simulink model "Sensing_Circuit_Test"  (R2020b)
settings: Solver=FixedStepAuto  StartTime=0.0  StopTime=10.0  FixedStep=1e-3  RelTol=1e-3  EnableMultiTasking=on
undefined symbols (not defined in the file): D0, D1, D13, D3, D6, PTA1, PTC16, PTC17, PTC2, PTD1
libraries: frdmk64flib x7
settings Model: ExtModeTrigDuration=5  Creator=Nour  LastModifiedBy=Nour
settings OptimizationCC: EnhancedBackFolding=on  PassReuseOutputArgsAs=Individual arguments  ZeroExternalMemoryAtStartup=off  ZeroInternalMemoryAtStartup=off  MaxStackSize=64  OptimizeBlockOrder=speed  DifferentSizesBufferReuse=on  OptimizationCustomize=off  EfficientTunableParamExpr=on
settings DebuggingCC: ParameterTunabilityLossMsg=error
settings HardwareCC: ProdBitPerPointer=32  ProdBitPerSizeT=32  ProdBitPerPtrDiffT=32  ProdLargestAtomicInteger=Long  ProdLargestAtomicFloat=Double  ProdWordSize=32  ProdHWDeviceType=ARM Compatible->ARM Cortex
settings SFSimCC: MATLABDynamicMemAlloc=off
settings RTWCC: Description=Embedded Coder  SystemTargetFile=ert.tlc  HardwareBoard=NXP FRDM-K64F  TLCOptions="-aInlineSetEventsForThisBaseRateFcn=TLC_FALSE -aSuppressMultiTaskScheduler=TLC_FALSE  -aRateBasedStepFcn=0"  TemplateMakefile=ert_default_tmf  Toolchain=GNU Tools for ARM Embedded Processors
settings CodeAppCC: ForceParamTrailComments=on  IgnoreCustomStorageClasses=off  OperatorAnnotations=on  SimulinkDataObjDesc=on  SFDataObjDesc=on  InsertBlockDesc=on
settings ERTTargetCC: ExtModeTransport=4  ExtModeMexFile=sendToCommService

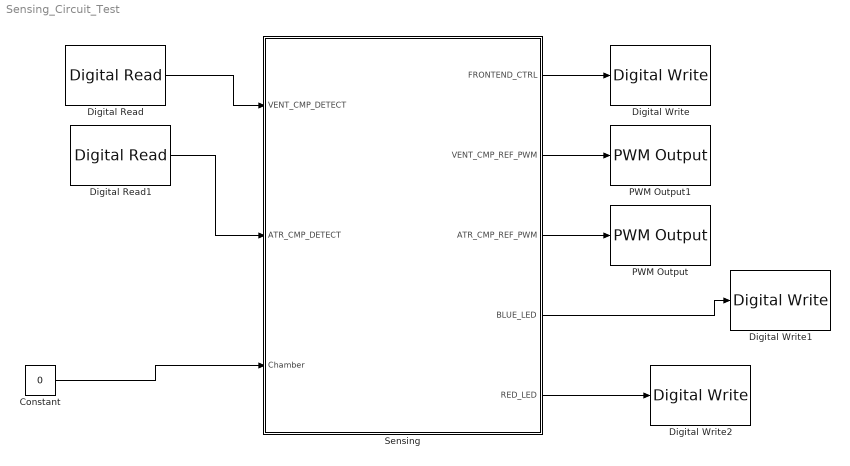
== system Sensing_Circuit_Test ==
  Constant : Constant  Value=0
  Digital Read : frdmk64flib/Digital Read  Whichpin=PTC17 (D1)  SampleTime=-1
  Digital Read1 : frdmk64flib/Digital Read  Whichpin=PTC16 (D0)  SampleTime=-1
  Digital Write : frdmk64flib/Digital Write  Whichpin=PTD1 (D13)
  Digital Write1 : frdmk64flib/Digital Write  Whichpin=BLUE_LED
  Digital Write2 : frdmk64flib/Digital Write  Whichpin=RED_LED
  PWM Output : frdmk64flib/PWM Output  Whichpin=PTC2 (D6)  InitialFrequency=2000  InitialDutyCycle=40
  PWM Output1 : frdmk64flib/PWM Output  Whichpin=PTA1 (D3)  InitialFrequency=2000  InitialDutyCycle=40
  Sensing : Stateflow chart  TreatAsAtomicUnit=on
  wires:
  Digital Read/1 -> Sensing/1(VENT_CMP_DETECT)
  Digital Read1/1 -> Sensing/2(ATR_CMP_DETECT)
  Sensing/1(FRONTEND_CTRL) -> Digital Write/1
  Sensing/2(VENT_CMP_REF_PWM) -> PWM Output1/1
  Sensing/3(ATR_CMP_REF_PWM) -> PWM Output/1
  Constant/1 -> Sensing/3(Chamber)
  Sensing/4(BLUE_LED) -> Digital Write1/1
  Sensing/5(RED_LED) -> Digital Write2/1

== stateflow chart Sensing_Circuit_Test/Sensing ==
  state ATR_DETECT
    entry:
    during:
    FRONTEND_CTRL = true;
    VENT_CMP_REF_PWM = 0;
    ATR_CMP_REF_PWM = 80;
    RED_LED = ATR_CMP_DETECT;
  state VENT_DETECT
    %% Chamber == 1 is for the Atrium
    %% Chamber == 0 is for the Ventricle
    entry:
    during:
    if(Chamber == 0)
    FRONTEND_CTRL = true;
    VENT_CMP_REF_PWM = 80;
    ATR_CMP_REF_PWM = 0;
    BLUE_LED = VENT_CMP_DETECT;
    end
    exit:
  (default) -> VENT_DETECT
  VENT_DETECT -> ATR_DETECT : [(Chamber == 1)]
  data: VENT_CMP_DETECT input boolean; ATR_CMP_DETECT input boolean; FRONTEND_CTRL output boolean; VENT_CMP_REF_PWM output int16; ATR_CMP_REF_PWM output int16; Chamber input double; BLUE_LED output boolean; RED_LED output boolean
